simulink model "InputsSimulated"  (R2018b)
settings: configuration reference "FixedStepConfiguration" (kept outside this file)
undefined symbols (not defined in the file): sigbuilder_block
settings Model: DataDictionary=DataDictionary.sldd  Creator=chris  LastModifiedBy=chris

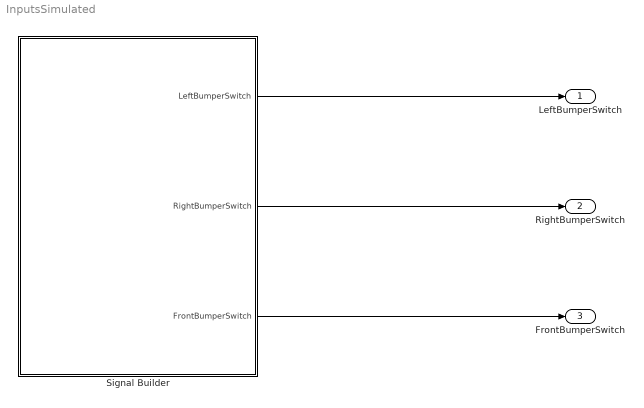
== system InputsSimulated ==
  Signal Builder : Subsystem  Tag=STV Subsys  LoadFcn=sigbuilder_block('load');  StartFcn=sigbuilder_block('start');  StopFcn=sigbuilder_block('stop');  ClipboardFcn=sigbuilder_block('clipboard');  mask(Sigbuilder block){tuvar=[0:10]}
      mask help: Simulink:masks:SigbuilderBlock_MD
      mask init:
      | if ~strcmp(get_param(bdroot(gcbh),'SimulationStatus'),'stopped') tuvar = sigbuilder_block('maskInit'); end
      settings: CopyFcn=sigbuilder_block('copy');  DeleteFcn=sigbuilder_block('delete');  ModelCloseFcn=sigbuilder_block('modelClose');  PreSaveFcn=sigbuilder_block('preSave');  PauseFcn=sigbuilder_block('pause');  ContinueFcn=sigbuilder_block('continue');  NameChangeFcn=sigbuilder_block('namechange');  OpenFcn=sigbuilder_block('open',[0.75 30.75 718.5 715.5 ]);  CloseFcn=sigbuilder_block('close');
      mask Display: plot(0, 0, 100, 100,[2, 2, 32, 32, 2], [68, 8, 8, 68, 68],[32, 2], [38, 38], [32, 19, 2],[53, 60, 44], [32, 17, 17, 2],[16, 16, 31, 31]);txt = getActiveGroup(gcbh);text(2, 100, txt,'verticalAlignment', 'top');
  LeftBumperSwitch : Outport
  RightBumperSwitch : Outport  Port=2
  FrontBumperSwitch : Outport  Port=3
  wires:
  Signal Builder/2(RightBumperSwitch) -> RightBumperSwitch/1
  Signal Builder/3(FrontBumperSwitch) -> FrontBumperSwitch/1
  Signal Builder/1(LeftBumperSwitch) -> LeftBumperSwitch/1

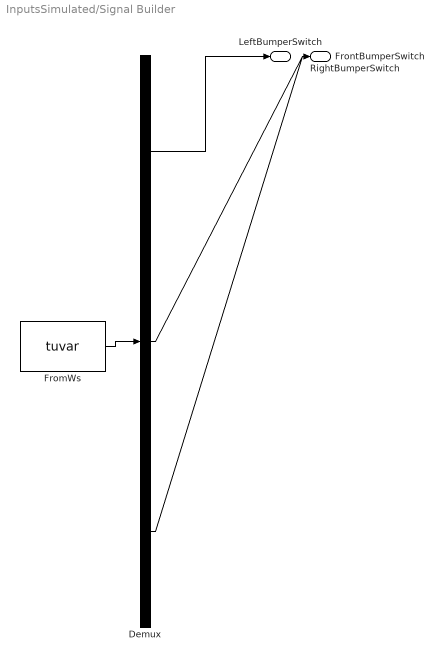
== system InputsSimulated/Signal Builder ==
  Demux : Demux  Tag=STV Demux  Outputs=3
  FromWs : FromWorkspace  Tag=STV FromWs  VariableName=tuvar  SampleTime=0
      SigBuilderData=|
      | common.afterFinalStr = 'Extrapolate'
      | common.sampleTime = 0
      | dataSet.timeRange = [0 30]
      | dataSet.name = 'Group 1'
      | sbobj.Groups.Name = 'Group 1'
      | sbobj.Groups.Signals(1).Name = 'LeftBumperSwitch'
      | sbobj.Groups.Signals(1).XData = [0 4 4 6 6 30]
      | sbobj.Groups.Signals(1).YData = [0 0 1 1 0 0]
      | sbobj.Groups.Signals(2).Name = 'RightBumperSwitch'
      | sbobj.Groups.Signals(2).XData = [0 12 12 18 18 30]
      | sbobj.Groups.Signals(2).YData = [0 0 1 1 0 0]
      | sbobj.Groups.Signals(3).Name = 'FrontBumperSwitch'
      | sbobj.Groups.Signals(3).XData = [0 20.9 20.9 25.45 25.45 30]
      | sbobj.Groups.Signals(3).YData = [0 0 1 1 0 0]
      | sbobj.Groups.TimeRange = [0 30]
  LeftBumperSwitch : Outport  Tag=STV Outport
  RightBumperSwitch : Outport  Tag=STV Outport  Port=2
  FrontBumperSwitch : Outport  Tag=STV Outport  Port=3
  wires:
  Demux/1 -> LeftBumperSwitch/1
  FromWs/1 -> Demux/1
  Demux/2 -> RightBumperSwitch/1
  Demux/3 -> FrontBumperSwitch/1
